simulink model "rev_3f_UW"  (Simulink 9.3)
settings: Solver=ode4  StartTime=0.0  StopTime=0.1  FixedStep=2e-4  MaxStep=2e-4  RelTol=1e-3  AbsTol=1e-6  EnableMultiTasking=on
libraries: powerlib x14, powerlib_extras x6
settings Model: Creator=Teacher  LastModifiedBy=ogure
settings SolverCC: AutoScaleAbsTol=off  SolverResetMethod=Robust
settings DataIOCC: SaveOutput=off  SaveTime=off
settings OptimizationCC: BlockReduction=off  BooleanDataType=off  InitFltsAndDblsToZero=on
settings DebuggingCC: SaveWithParameterizedLinksMsg=none  SignalResolutionControl=TryResolveAllWithWarning  MultiTaskDSMMsg=warning  MultiTaskCondExecSysMsg=none
settings HardwareCC: TargetHWDeviceType=32-bit Generic
settings GRTTargetCC: TargetFcnLib=ansi_tfl_tmw.mat  GeneratePreprocessorConditionals=Disable all
settings ConfigComp: CovSFcnEnable=off
settings SimscapeCC: SimscapeNormalizeSystem=off

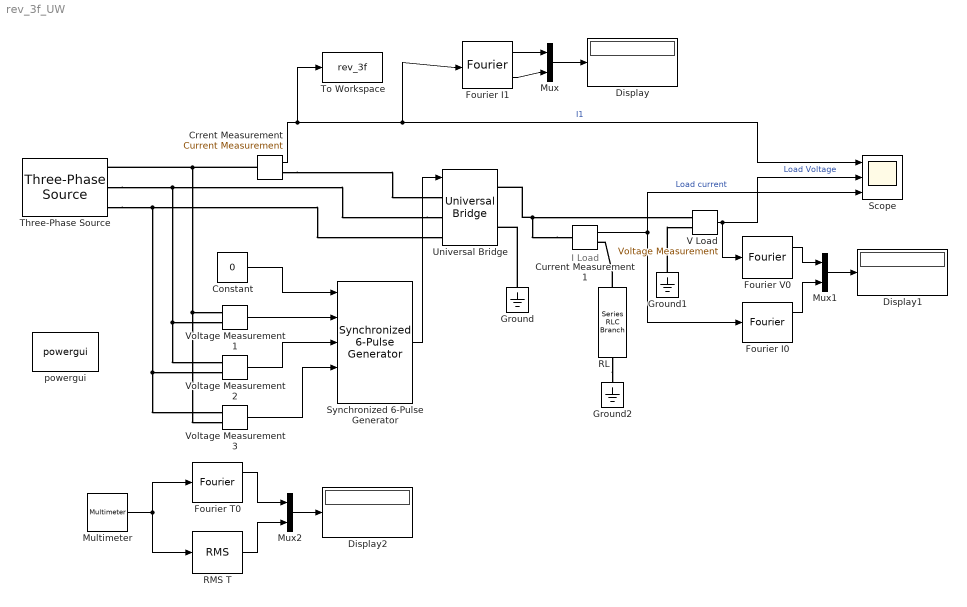
== system rev_3f_UW ==
  note: I Load
  Constant : Constant  Value=0  VectorParams1D=off
  Crrent Measurement : powerlib/Measurements/Current Measurement  Tag=PoWeRsYsTeMmEaSuReMeNt  PhasorSimulation=off  OutputType=Complex  PSBequivalent=0
      settings: SourceProductName=Simscape Electrical
  Current Measurement1 : powerlib/Measurements/Current Measurement  PhasorSimulation=off  OutputType=Complex  PSBequivalent=0
      settings: SourceProductName=Simscape Electrical
  Display : Display
      settings: SampleTime=2e-4
  Display1 : Display
      settings: SampleTime=2e-4
  Display2 : Display
      settings: SampleTime=2e-4
  Fourier I0 : powerlib_extras/Measurements/Fourier  f1=300  n=0
      settings: SourceProductName=Simscape Electrical  SourceProductBaseCode=PS
  Fourier I1 : powerlib_extras/Measurements/Fourier  f1=50  n=1
      settings: SourceProductName=Simscape Electrical  SourceProductBaseCode=PS
  Fourier T0 : powerlib_extras/Measurements/Fourier  f1=300  n=0
      settings: SourceProductName=Simscape Electrical  SourceProductBaseCode=PS
  Fourier V0 : powerlib_extras/Measurements/Fourier  f1=300  n=0
      settings: SourceProductName=Simscape Electrical  SourceProductBaseCode=PS
  Ground : powerlib/Elements/Ground  LConnTagsString=a
      settings: SourceProductName=Simscape Electrical
  Ground1 : powerlib/Elements/Ground  LConnTagsString=a
      settings: SourceProductName=Simscape Electrical
  Ground2 : powerlib/Elements/Ground  LConnTagsString=a
      settings: SourceProductName=Simscape Electrical
  Multimeter : powerlib/Measurements/Multimeter  PhasorSimulation=off  OutputType=Complex  sel=[11 1]  L=16  Gain=[1 1]  yselected={'Isw1: Universal Bridge','Usw1: Universal Bridge'};  PSBOutputType=1  PSBequivalent=0  AxesSetting=[0,0.1,-100,100]  Display=1  SavedBlockNames=-11
      settings: SourceProductName=Simscape Electrical
  Mux : Mux  Inputs=2
  Mux1 : Mux  Inputs=2
  Mux2 : Mux  Inputs=2
  RL : powerlib/Elements/Series RLC Branch  LConnTagsString=__new0  RConnTagsString=__new0  BranchType=RL  Resistance=0.04  Inductance=530.5e-6  SetiL0=off  InitialCurrent=0  Capacitance=inf  Setx0=off  InitialVoltage=0  Measurements=None
      settings: SourceProductName=Simscape Electrical
  RMS T : powerlib_extras/Measurements/RMS  f1=60
      settings: SourceProductName=Simscape Electrical  SourceProductBaseCode=PS
  Scope : Scope  NumInputPorts=3
  Synchronized 6-Pulse Generator : powerlib_extras/Control  Blocks/Synchronized 6-Pulse Generator  freq=50  pwidth=10  Double_Pulse=off
      settings: SourceProductName=Simscape Electrical  SourceProductBaseCode=PS
  Three-Phase Source : powerlib/Electrical Sources/Three-Phase Source  InternalConnection=Yn  VoltagePhases=off  Voltage=9.2*sqrt(3)  PhaseAngle=0  Voltage_phases=[25e3 25e3 25e3]/sqrt(3)  PhaseAngles_phases=[0 -120 +120]  Frequency=50  NonIdealSource=on  SpecifyImpedance=off  Resistance=0.69  Inductance=0  ShortCircuitLevel=100e6  BaseVoltage=25e4  XRratio=7  BusType=swing  Pref=0  Qref=0  Prefabc=[10e3, 10e3, 10e3]  Qrefabc=[0, 0, 0]  Qmin=-inf  Qmax=inf
      settings: SourceProductName=Simscape Electrical
  To Workspace : ToWorkspace  VariableName=rev_3f  SampleTime=2e-4
      settings: MaxDataPoints=200
  Universal Bridge : powerlib/Power Electronics/Universal Bridge  Arms=3  SnubberResistance=1e6  SnubberCapacitance=1e-9  Device=Thyristors  Ron=1.05e-3  Lon=0  ForwardVoltages="[  0  0  ]"  ForwardVoltage=1.05  GTOparameters=[ 10e-6 , 20e-6 ]  IGBTparameters=[ 1e-6 , 2e-6 ]  Measurements=All voltages and currents  Measurements_2=None  converterType=Rectifier
      settings: SourceProductName=Simscape Electrical
  V Load : powerlib/Measurements/Voltage Measurement  PhasorSimulation=off  OutputType=Complex  PSBequivalent=0
      settings: SourceProductName=Simscape Electrical
  Voltage Measurement1 : powerlib/Measurements/Voltage Measurement  PhasorSimulation=off  OutputType=Complex  PSBequivalent=0
      settings: SourceProductName=Simscape Electrical
  Voltage Measurement2 : powerlib/Measurements/Voltage Measurement  PhasorSimulation=off  OutputType=Complex  PSBequivalent=0
      settings: SourceProductName=Simscape Electrical
  Voltage Measurement3 : powerlib/Measurements/Voltage Measurement  PhasorSimulation=off  OutputType=Complex  PSBequivalent=0
      settings: SourceProductName=Simscape Electrical
  powergui : powerlib/powergui  Priority=1  SimulationMode=Continuous  SampleTime=2e-4  frequency=60  Iterations=50  frequencyindice=50  Pbase=100e6  ErrMax=1e-4  UnitsV=kV  UnitsW=MW  buscounter=0  FunctionMessages=off  echomessages=off  EnableUseOfTLC=off  CurrentSourceSwitches=off  DisableSnubberDevices=off  DisableRonSwitches=off  DisableVfSwitches=off  DisplayEquations=off  AutomaticDiscreteSolvers=off  SolverType=Tustin/Backward Euler (TBE)  Interpol=off  ExternalGateDelay=off  methode=off  Ts=100  x0status=blocks  SPID=off  SwTol=0  HookPort=off  NonlinearTolerance=0  nMaxIteration=15  ContinueOnMaxIteration=off  RestoreLinks=warning  ResistiveCurrentMeasurement=off  Frange=[0:2:500]  Ylog=off  Xlog=on  ShowGrid=off  save=off  variable=ZData  structure=0  ZoomFFT=off  StartTime=0.0  cycles=1  DisplayStyle=1  fundamental=60  FreqAxis=off  MaxFrequency=1000  frequencyindicesteady=1  RmsSteady=1  display=off
      settings: SourceProductName=Simscape Electrical
  wires:
  Fourier I1/1 -> Mux/1
  Fourier I1/2 -> Mux/2
  Fourier I0/1 -> Mux1/2
  Fourier V0/1 -> Mux1/1
  V Load/1 -> Fourier V0/1, Scope/2  "Load Voltage"
  Current Measurement1/1 -> Fourier I0/1, Scope/3  "Load current"
  Mux1/1 -> Display1/1
  Mux/1 -> Display/1
  Voltage Measurement1/1 -> Synchronized 6-Pulse Generator/2
  Voltage Measurement2/1 -> Synchronized 6-Pulse Generator/3
  Voltage Measurement3/1 -> Synchronized 6-Pulse Generator/4
  Constant/1 -> Synchronized 6-Pulse Generator/1
  Synchronized 6-Pulse Generator/1 -> Universal Bridge/1
  Crrent Measurement/1 -> Fourier I1/1, Scope/1, To Workspace/1  "I1"
  Multimeter/1 -> Fourier T0/1, RMS T/1
  Mux2/1 -> Display2/1
  Fourier T0/1 -> Mux2/1
  RMS T/1 -> Mux2/2
  connections:
  Crrent Measurement/RConn1 -- Universal Bridge/LConn1
  Current Measurement1/LConn1 -- Universal Bridge/RConn1 -- V Load/LConn1
  RL/LConn1 -- Current Measurement1/RConn1
  Ground/LConn1 -- Universal Bridge/RConn2
  Ground1/LConn1 -- V Load/LConn2
  Crrent Measurement/LConn1 -- Three-Phase Source/RConn1 -- Voltage Measurement3/LConn2 -- Voltage Measurement1/LConn1
  Universal Bridge/LConn2 -- Three-Phase Source/RConn2 -- Voltage Measurement2/LConn1 -- Voltage Measurement1/LConn2
  Three-Phase Source/RConn3 -- Universal Bridge/LConn3 -- Voltage Measurement3/LConn1 -- Voltage Measurement2/LConn2
  RL/RConn1 -- Ground2/LConn1
